simulink model "admittance"  (R2021b)
settings: Solver=VariableStepAuto  StartTime=0.0  StopTime=5  RelTol=1e-3
undefined symbols (not defined in the file): K, Kd, KDt, Kp, KPt, Mt, xr
libraries: robotcorelib x1, simulink x1
settings Model: Creator=fabio  LastModifiedBy=buse
settings SolverCC: MaxConsecutiveMinStep=10

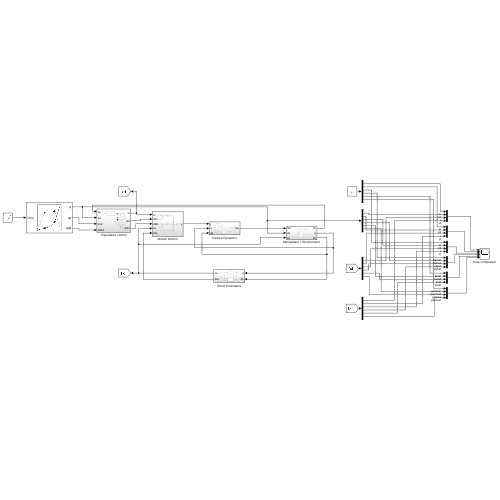
[thumbnail: Simulink's stored preview of the top-level diagram]
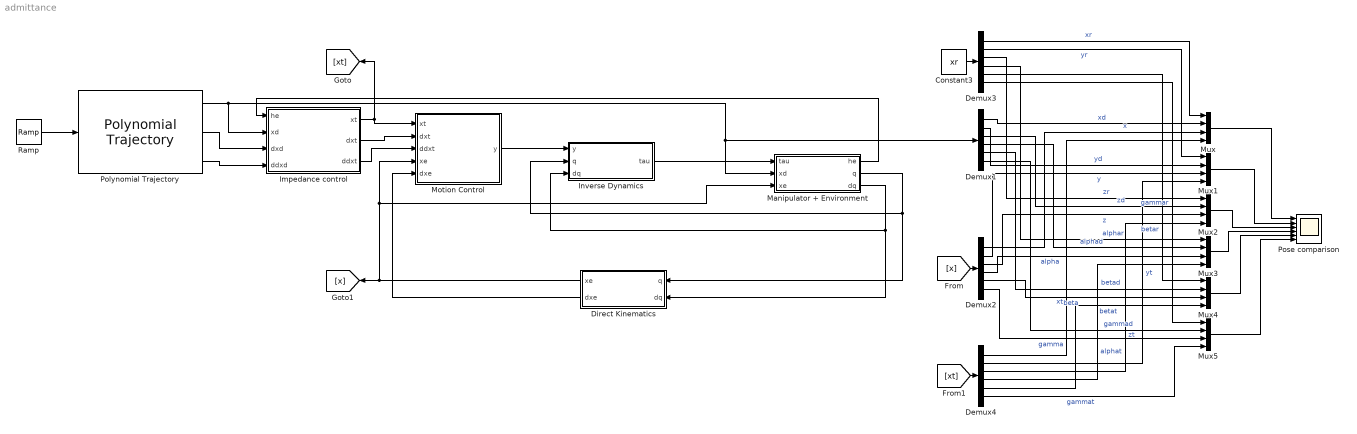
== system admittance ==
  Constant3 : Constant  Value=xr
  Demux{1..4} (4 alike) : Demux  Outputs=6
  Direct Kinematics : Subsystem
  Impedance control : Subsystem
  Inverse Dynamics : Subsystem
  Manipulator + Environment : Subsystem
  Motion Control : Subsystem
  Mux{,1..5} (6 alike) : Mux
  Polynomial Trajectory : robotcorelib/Polynomial Trajectory  WaypointSource=Internal  Waypoints=op_wpts  TimePoints=time  TimeInterval=[ 1, 4 ]  Method=Quintic Polynomial  ParameterSource=Internal  VelocityBoundaryCondition=velBound  AccelerationBoundaryCondition=accBound  SimulateUsing=Interpreted execution
  Pose comparison : Scope  NumInputPorts=6
  Ramp : simulink/Sources/Ramp  slope=1  start=0  InitialOutput=0
  wires:
  Mux1/1 -> Pose comparison/2
  Demux1/4 -> Mux3/2  "alphad"
  Demux1/1 -> Mux/2  "xd"
  Mux4/1 -> Pose comparison/5
  Demux2/1 -> Mux/3  "x"
  Demux1/3 -> Mux2/2  "zd"
  Demux2/4 -> Mux3/3  "alpha"
  Demux1/6 -> Mux5/2  "gammad"
  Demux2/2 -> Mux1/3  "y"
  Mux/1 -> Pose comparison/1
  Demux2/3 -> Mux2/3  "z"
  Polynomial Trajectory/1 -> Impedance control/2(xd), Demux1/1, Manipulator + Environment/2(xd)
  Mux3/1 -> Pose comparison/4
  Demux2/5 -> Mux4/3  "beta"
  Demux1/2 -> Mux1/2  "yd"
  Demux1/5 -> Mux4/2  "betad"
  Mux5/1 -> Pose comparison/6
  Mux2/1 -> Pose comparison/3
  [x] -> Demux2/1
  Demux2/6 -> Mux5/3  "gamma"
  Constant3/1 -> Demux3/1
  Demux3/1 -> Mux/1  "xr"
  Demux3/2 -> Mux1/1  "yr"
  Demux3/3 -> Mux2/1  "zr"
  Demux3/4 -> Mux3/1  "alphar"
  Demux3/5 -> Mux4/1  "betar"
  Demux3/6 -> Mux5/1  "gammar"
  Manipulator + Environment/2(q) -> Inverse Dynamics/2(q), Direct Kinematics/1(q)
  Direct Kinematics/1(xe) -> Motion Control/4(xe), Manipulator + Environment/3(xe), [x]
  Motion Control/1(y) -> Inverse Dynamics/1(y)
  Inverse Dynamics/1(tau) -> Manipulator + Environment/1(tau)
  Manipulator + Environment/3(dq) -> Direct Kinematics/2(dq), Inverse Dynamics/3(dq)
  Ramp/1 -> Polynomial Trajectory/1
  Impedance control/1(xt) -> [xt], Motion Control/1(xt)
  Polynomial Trajectory/3 -> Impedance control/4(ddxd)
  Polynomial Trajectory/2 -> Impedance control/3(dxd)
  Manipulator + Environment/1(he) -> Impedance control/1(he)
  Impedance control/2(dxt) -> Motion Control/2(dxt)
  Impedance control/3(ddxt) -> Motion Control/3(ddxt)
  Direct Kinematics/2(dxe) -> Motion Control/5(dxe)
  [xt] -> Demux4/1
  Demux4/1 -> Mux/4  "xt"
  Demux4/2 -> Mux1/4  "yt"
  Demux4/3 -> Mux2/4  "zt"
  Demux4/4 -> Mux3/4  "alphat"
  Demux4/5 -> Mux4/4  "betat"
  Demux4/6 -> Mux5/4  "gammat"

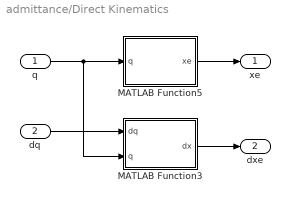
== system admittance/Direct Kinematics ==
  q : Inport
  dq : Inport  Port=2
  MATLAB Function3 : MATLAB Function  TreatAsAtomicUnit=on
  MATLAB Function5 : MATLAB Function  TreatAsAtomicUnit=on
  xe : Outport
  dxe : Outport  Port=2
  wires:
  MATLAB Function3/1(dx) -> dxe/1
  q/1 -> MATLAB Function3/2(q), MATLAB Function5/1(q)
  MATLAB Function5/1(xe) -> xe/1
  dq/1 -> MATLAB Function3/1(dq)

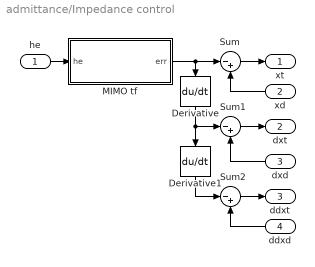
== system admittance/Impedance control ==
  he : Inport
  xd : Inport  Port=2
  dxd : Inport  Port=3
  ddxd : Inport  Port=4
  Derivative : Derivative
  Derivative1 : Derivative
  MIMO tf : Subsystem
  Sum : Sum  Inputs=|-+
  Sum1 : Sum  Inputs=|-+
  Sum2 : Sum  Inputs=|-+
  xt : Outport
  dxt : Outport  Port=2
  ddxt : Outport  Port=3
  wires:
  xd/1 -> Sum/2
  Sum/1 -> xt/1
  he/1 -> MIMO tf/1(he)
  MIMO tf/1(err) -> Derivative/1, Sum/1
  dxd/1 -> Sum1/2
  Sum1/1 -> dxt/1
  Derivative/1 -> Sum1/1, Derivative1/1
  ddxd/1 -> Sum2/2
  Sum2/1 -> ddxt/1
  Derivative1/1 -> Sum2/1

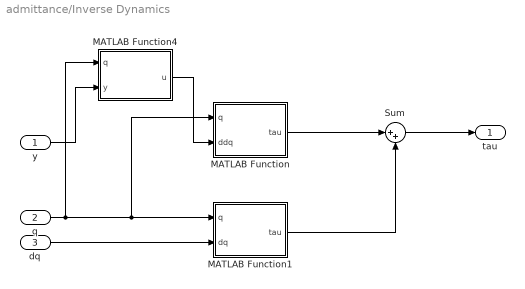
== system admittance/Inverse Dynamics ==
  y : Inport
  q : Inport  Port=2
  dq : Inport  Port=3
  MATLAB Function : MATLAB Function  TreatAsAtomicUnit=on
  MATLAB Function1 : MATLAB Function  TreatAsAtomicUnit=on
  MATLAB Function4 : MATLAB Function  TreatAsAtomicUnit=on
  Sum : Sum  Inputs=|++
  tau : Outport
  wires:
  MATLAB Function1/1(tau) -> Sum/2
  MATLAB Function/1(tau) -> Sum/1
  Sum/1 -> tau/1
  dq/1 -> MATLAB Function1/2(dq)
  q/1 -> MATLAB Function4/1(q), MATLAB Function/1(q), MATLAB Function1/1(q)
  MATLAB Function4/1(u) -> MATLAB Function/2(ddq)
  y/1 -> MATLAB Function4/2(y)

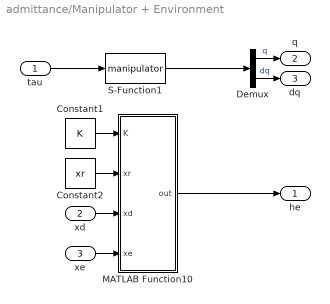
== system admittance/Manipulator + Environment ==
  tau : Inport
  xd : Inport  Port=2
  xe : Inport  Port=3
  Constant1 : Constant  Value=K
  Constant2 : Constant  Value=xr
  Demux : Demux  Outputs=2
  MATLAB Function10 : MATLAB Function  TreatAsAtomicUnit=on
  S-Function1 : S-Function  FunctionName=manipulator  Parameters=robot  SFunctionDeploymentMode=off  EnableBusSupport=off
  he : Outport
  q : Outport  Port=2
  dq : Outport  Port=3
  wires:
  tau/1 -> S-Function1/1
  Constant1/1 -> MATLAB Function10/1(K)
  Constant2/1 -> MATLAB Function10/2(xr)
  xd/1 -> MATLAB Function10/3(xd)
  xe/1 -> MATLAB Function10/4(xe)
  S-Function1/1 -> Demux/1
  Demux/1 -> q/1  "q"
  Demux/2 -> dq/1  "dq"
  MATLAB Function10/1(out) -> he/1

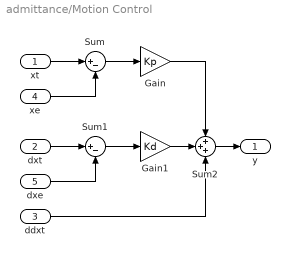
== system admittance/Motion Control ==
  xt : Inport
  dxt : Inport  Port=2
  ddxt : Inport  Port=3
  xe : Inport  Port=4
  dxe : Inport  Port=5
  Gain : Gain  Gain=Kp
  Gain1 : Gain  Gain=Kd
  Sum : Sum  Inputs=|+-
  Sum1 : Sum  Inputs=|+-
  Sum2 : Sum  Inputs=+++
  y : Outport
  wires:
  xt/1 -> Sum/1
  xe/1 -> Sum/2
  Sum/1 -> Gain/1
  dxt/1 -> Sum1/1
  dxe/1 -> Sum1/2
  Sum1/1 -> Gain1/1
  Gain/1 -> Sum2/1
  Gain1/1 -> Sum2/2
  Sum2/1 -> y/1
  ddxt/1 -> Sum2/3

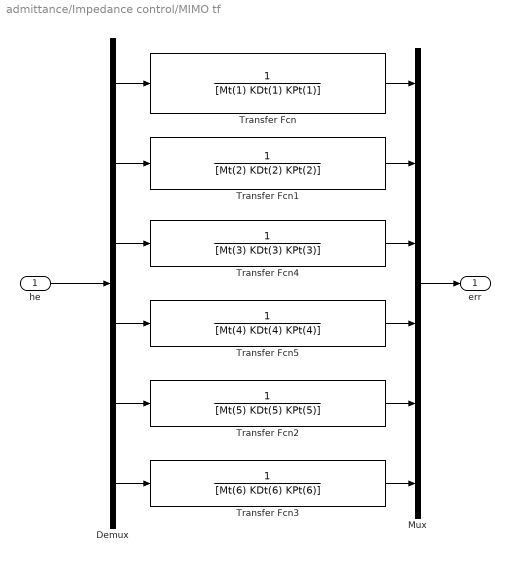
== system admittance/Impedance control/MIMO tf ==
  he : Inport
  Demux : Demux  Outputs=6
  Mux : Mux  Inputs=6
  Transfer Fcn : TransferFcn  Denominator=[Mt(1) KDt(1) KPt(1)]
  Transfer Fcn1 : TransferFcn  Denominator=[Mt(2) KDt(2) KPt(2)]
  Transfer Fcn2 : TransferFcn  Denominator=[Mt(5) KDt(5) KPt(5)]
  Transfer Fcn3 : TransferFcn  Denominator=[Mt(6) KDt(6) KPt(6)]
  Transfer Fcn4 : TransferFcn  Denominator=[Mt(3) KDt(3) KPt(3)]
  Transfer Fcn5 : TransferFcn  Denominator=[Mt(4) KDt(4) KPt(4)]
  err : Outport
  wires:
  Demux/4 -> Transfer Fcn5/1
  Transfer Fcn5/1 -> Mux/4
  Transfer Fcn3/1 -> Mux/6
  Transfer Fcn1/1 -> Mux/2
  Transfer Fcn2/1 -> Mux/5
  Mux/1 -> err/1
  Demux/3 -> Transfer Fcn4/1
  Demux/6 -> Transfer Fcn3/1
  Demux/2 -> Transfer Fcn1/1
  he/1 -> Demux/1
  Transfer Fcn/1 -> Mux/1
  Demux/1 -> Transfer Fcn/1
  Transfer Fcn4/1 -> Mux/3
  Demux/5 -> Transfer Fcn2/1

== matlab function admittance/Inverse Dynamics/MATLAB Function1 ==
  data: q input size=3; tau output; dq input size=3
function tau = N(q, dq)
    q1 = q(1); q2 = q(2); q3 = q(3);
    dq1 = dq(1); dq2 = dq(2); dq3 = dq(3);
    tau = [dq3*(0.03923*cos(q3)*dq3^2 - 0.5*dq1*(0.0474*sin(2.0*q3) + 0.05885*sin(q3) + 0.1962*q2*sin(q3))*dq3) - 1.0*dq1*(0.5*dq3^2*(0.0474*sin(2.0*q3) + 0.05885*sin(q3) + 0.1962*q2*sin(q3)) - 0.5*dq2^2*(3.098*q2 + 0.1962*cos(q3) + 0.7099)) + 0.5*dq1*dq2^2*(3.098*q2 + 0.1962*cos(q3) + 0.7099);
            0.5*dq1^2*dq2*(3.098*q2 + 0.1962*cos(q3) + 0.7099);
            dq1*(0.03923*cos(q3)*dq3^2 - 0.5*dq1*(0.0474*sin(2.0*q3) + 0.05885*sin(q3) + 0.1962*q2*sin(q3))*dq3) - 0.9621*cos(q3)];
end

== matlab function admittance/Inverse Dynamics/MATLAB Function ==
  data: q input size=3; tau output; ddq input size=3
function tau = B(q, ddq)
    q1 = q(1); q2 = q(2); q3 = q(3);
    B = getB(q,0);
    tau = B*ddq;

== matlab function admittance/Direct Kinematics/MATLAB Function3 ==
  data: dq input; dx output; q input
function dx = JA(dq, q)
    q1 = q(1); q2 = q(2); q3 = q(3);
    JA =[(3*cos(q1))/10 - (2*sin(q1))/5 + (6*cos(q1)*cos(q3))/25 + q2*cos(q1),  sin(q1), -(6*sin(q1)*sin(q3))/25;
        (2*cos(q1))/5 + (3*sin(q1))/10 + (6*cos(q3)*sin(q1))/25 + q2*sin(q1), -cos(q1),  (6*cos(q1)*sin(q3))/25;
        0,        0,          (6*cos(q3))/25;
        1,        0,                       0;
        0,        0,                      -1;
        0,        0,                       0]; 
    dx = JA*dq;

== matlab function admittance/Inverse Dynamics/MATLAB Function4 ==
  data: q input; y input; u output
function u = invJA(q,y)
    q1 = q(1); q2 = q(2); q3 = q(3);
    JAinv =  [
[                                                                                                                                                             (10.0*cos(q1)*(1.0e+33*q2 + 2.4e+32*cos(q3) + 3.0e+32))/(6.0e+33*q2 + 1.44e+33*cos(q3) + 5.76e+32*cos(q3)^2 + 4.8e+33*q2*cos(q3) + 1.0e+34*q2^2 + 1.09e+34),                                                                                                                                                                         (10.0*sin(q1)*(1.0e+33*q2 + 2.4e+32*cos(q3) + 3.0e+32))/(6.0e+33*q2 + 1.44e+33*cos(q3) + 5.76e+32*cos(q3)^2 + 4.8e+33*q2*cos(q3) + 1.0e+34*q2^2 + 1.09e+34),                                                         0, 1.0e+34/(6.0e+33*q2 + 1.44e+33*cos(q3) + 5.76e+32*cos(q3)^2 + 4.8e+33*q2*cos(q3) + 1.0e+34*q2^2 + 1.09e+34),                                                  0, 0]
[(1.2e+33*cos(q1) + 1.09e+34*sin(q1) + 9.6e+32*cos(q1)*cos(q3) + 1.0e+34*q2^2*sin(q1) + 1.44e+33*cos(q3)*sin(q1) + 5.76e+32*cos(q3)^2*sin(q1) + 4.0e+33*q2*cos(q1) + 6.0e+33*q2*sin(q1) + 4.8e+33*q2*cos(q3)*sin(q1))/(6.0e+33*q2 + 1.44e+33*cos(q3) + 5.76e+32*cos(q3)^2 + 4.8e+33*q2*cos(q3) + 1.0e+34*q2^2 + 1.09e+34), -(1.0e-32*(1.09e+66*cos(q1) - 1.2e+65*sin(q1) + 1.0e+66*q2^2*cos(q1) + 1.44e+65*cos(q1)*cos(q3) - 9.6e+64*cos(q3)*sin(q1) + 5.76e+64*cos(q1)*cos(q3)^2 + 6.0e+65*q2*cos(q1) - 4.0e+65*q2*sin(q1) + 4.8e+65*q2*cos(q1)*cos(q3)))/(6.0e+33*q2 + 1.44e+33*cos(q3) + 5.76e+32*cos(q3)^2 + 4.8e+33*q2*cos(q3) + 1.0e+34*q2^2 + 1.09e+34), (2.88e+32*sin(2.0*q3))/(2.88e+32*cos(2.0*q3) + 1.029e+34), 4.0e+33/(6.0e+33*q2 + 1.44e+33*cos(q3) + 5.76e+32*cos(q3)^2 + 4.8e+33*q2*cos(q3) + 1.0e+34*q2^2 + 1.09e+34), (2.4e+33*sin(q3))/(5.76e+32*sin(q3)^2 - 1.058e+34), 0]
[                                                                                                                                                                                                                                                                                                                       0,                                                                                                                                                                                                                                                                                                                                   0,          (2.4e+33*cos(q3))/(5.76e+32*cos(q3)^2 + 1.0e+34),                                                                                                           0,           1.0e+34/(5.76e+32*sin(q3)^2 - 1.058e+34), 0]];
    u = JAinv*y;

== matlab function admittance/Direct Kinematics/MATLAB Function5 ==
  data: q input size=3; xe output size=6
function xe = k(q)
    q1 = q(1); q2 = q(2); q3 = q(3);
    % Direct kinematics
    xe = [(2*cos(q1))/5 + (3*sin(q1))/10 + (6*cos(q3)*sin(q1))/25 + q2*sin(q1);
         (2*sin(q1))/5 - (3*cos(q1))/10 - (6*cos(q1)*cos(q3))/25 - q2*cos(q1);
         (6*sin(q3))/25 + 3/20;
         q1;
         pi/2 - q3;
         pi/2];

== matlab function admittance/Manipulator + Environment/MATLAB Function10 ==
  data: K input; out output size=6; xr input; xd input; xe input size=6
function out = he(K, xr, xd, xe)
    he = zeros(6,1);
    if xe(2) > xr(2) % Only along y, i.e. only when moving only joint 2
        % In contact
        dxrd = xd-xr;
        dxed = xd-xe;
        dxre = dxrd-dxed;
        he = K*dxre;
    end
    % Equilibrium point
    out = he;
